simulink model "CommsInMAV"  (R2026a)
settings: Solver=VariableStepAuto
libraries: simulink x3, uavmavlinklib x1
settings Model: DataDictionary=QuadData.sldd  Creator=The MathWorks, Inc.  LastModifiedBy=The MathWorks, Inc.

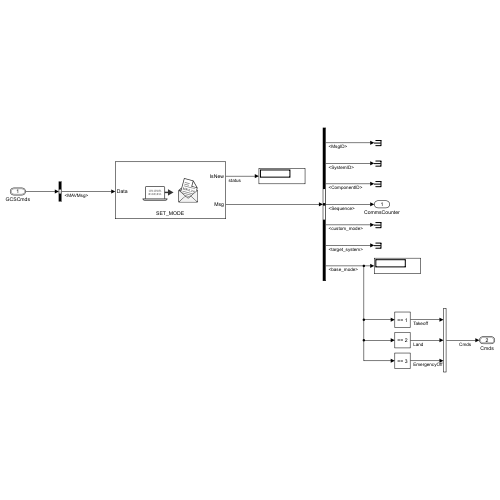
[thumbnail: Simulink's stored preview of the top-level diagram]
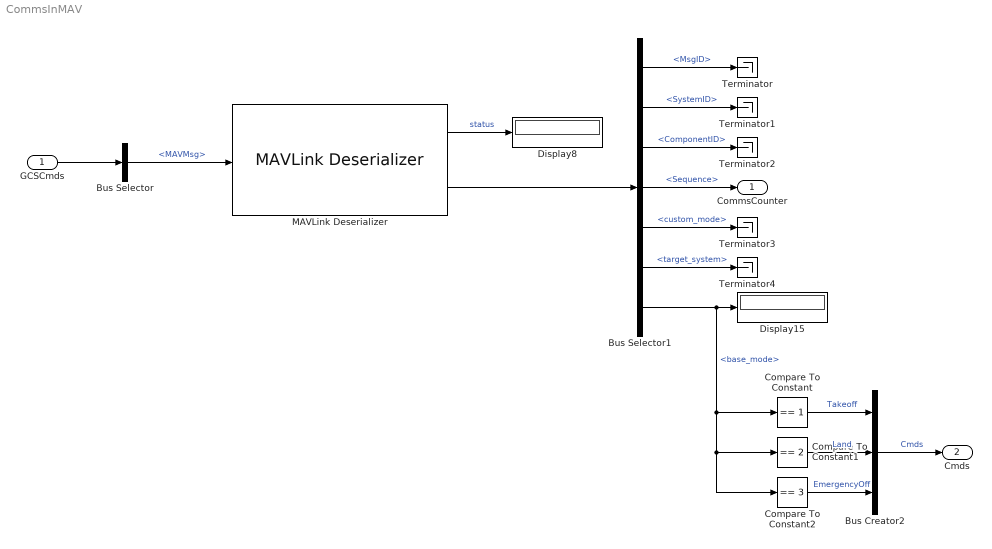
== system CommsInMAV ==
  GCSCmds : Inport  OutDataTypeStr=Bus: GCSCmds  BusOutputAsStruct=on
  Bus Creator2 : BusCreator  Inputs=3  OutDataTypeStr=Bus: Cmds  NonVirtualBus=on
  Bus Selector : BusSelector  OutputSignals=MAVMsg
  Bus Selector1 : BusSelector  OutputSignals=MsgID,SystemID,ComponentID,Sequence,Payload.custom_mode,Payload.target_system,Payload.base_mode
  Compare To Constant : simulink/Logic and Bit Operations/Compare To Constant  relop===  const=1  OutDataTypeStr=boolean  ZeroCross=off
  Compare To Constant1 : simulink/Logic and Bit Operations/Compare To Constant  relop===  const=2  OutDataTypeStr=boolean  ZeroCross=off
  Compare To Constant2 : simulink/Logic and Bit Operations/Compare To Constant  relop===  const=3  OutDataTypeStr=boolean  ZeroCross=off
  Display15 : Display
  Display8 : Display
  MAVLink Deserializer : uavmavlinklib/MAVLink Deserializer  dialectSource=Select from standard MAVLink dialects  dialect=common.xml  dialectCustom=common.xml  version=2  messageType=SET_MODE  inputDataLength=off  SystemIDFilter=off  systemID=1  ComponentIDFilter=off  componentID=1  queueMsg=off  queueMsgSize=50  dropNum=off
  Terminator{,1..4} (5 alike) : Terminator
  CommsCounter : Outport  OutDataTypeStr=uint8  PortDimensions=1  VectorParamsAs1DForOutWhenUnconnected=off
  Cmds : Outport  Port=2  OutDataTypeStr=Bus: Cmds
  wires:
  MAVLink Deserializer/2 -> Bus Selector1/1
  MAVLink Deserializer/1 -> Display8/1  "status"
  Bus Selector1/6 -> Terminator4/1  "<target_system>"
  Bus Selector1/2 -> Terminator1/1  "<SystemID>"
  Bus Selector1/5 -> Terminator3/1  "<custom_mode>"
  Bus Selector1/4 -> CommsCounter/1  "<Sequence>"
  Bus Selector1/7 -> Compare To Constant2/1, Compare To Constant1/1, Compare To Constant/1, Display15/1  "<base_mode>"
  Bus Selector1/1 -> Terminator/1  "<MsgID>"
  Bus Selector1/3 -> Terminator2/1  "<ComponentID>"
  Compare To Constant1/1 -> Bus Creator2/2  "Land"
  Compare To Constant/1 -> Bus Creator2/1  "Takeoff"
  Bus Creator2/1 -> Cmds/1  "Cmds"
  Compare To Constant2/1 -> Bus Creator2/3  "EmergencyOff"
  GCSCmds/1 -> Bus Selector/1
  Bus Selector/1 -> MAVLink Deserializer/1  "<MAVMsg>"
